simulink model "a2e1"  (R2020a)
settings: Solver=VariableStepAuto  StartTime=0.0  StopTime=400000  RelTol=1e-3
settings Model: EnablePacing=on  PacingRate=6  Creator=mumun  LastModifiedBy=mumun

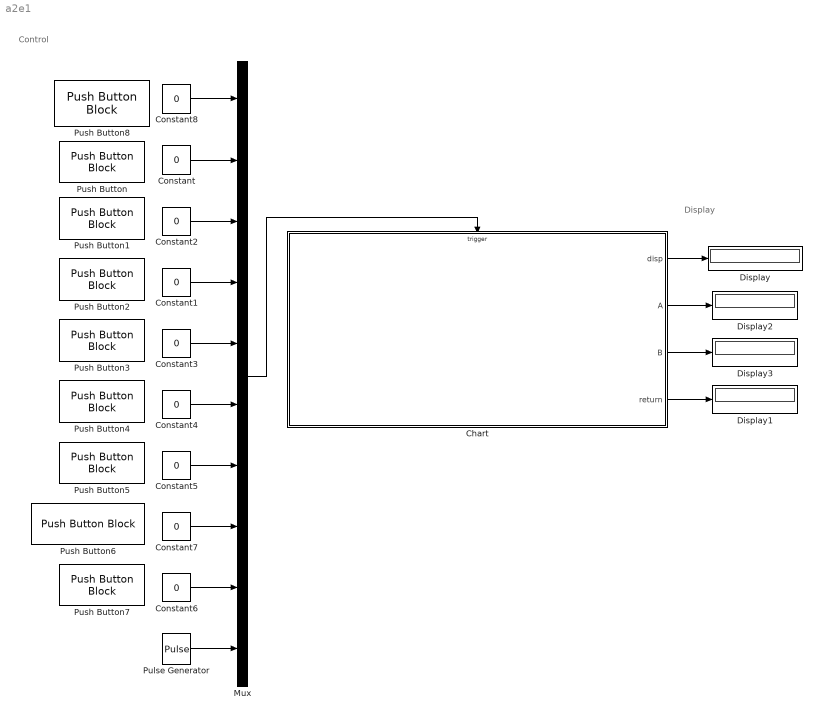
== system a2e1 ==
  note: Display
  note: Control
  Chart : Stateflow chart  TreatAsAtomicUnit=on
  Constant{,1..8} (9 alike) : Constant  Value=0
  Display{,1..3} (4 alike) : Display
  Mux : Mux  Inputs=10
  Pulse Generator : DiscretePulseGenerator  PulseType=Time based  Period=1  PulseWidth=5
  Push Button : PushButtonBlock  ButtonText=1kr
  Push Button1 : PushButtonBlock  ButtonText=5kr
  Push Button2 : PushButtonBlock  ButtonText=10kr
  Push Button3 : PushButtonBlock  ButtonText=order
  Push Button4 : PushButtonBlock  ButtonText=option_A
  Push Button5 : PushButtonBlock  ButtonText=option_B
  Push Button6 : PushButtonBlock  ButtonText=insert_more_money
  Push Button7 : PushButtonBlock  ButtonText=finish
  Push Button8 : PushButtonBlock  ButtonText=Start_Button
  wires:
  Mux/1 -> Chart/Trigger
  Chart/1(disp) -> Display/1
  Constant8/1 -> Mux/1
  Constant/1 -> Mux/2
  Constant2/1 -> Mux/3
  Constant1/1 -> Mux/4
  Constant3/1 -> Mux/5
  Constant4/1 -> Mux/6
  Constant5/1 -> Mux/7
  Constant7/1 -> Mux/8
  Constant6/1 -> Mux/9
  Chart/3(B) -> Display3/1
  Pulse Generator/1 -> Mux/10
  Chart/4(return) -> Display1/1
  Chart/2(A) -> Display2/1

== stateflow chart a2e1/Chart ==
  settings: executeAtInitialization=1  initializeOutput=1
  state coininsert
    du: disp= 'Insert coin';
    on one_kr: coin_count=coin_count+1;
    on five_kr: coin_count=coin_count+5;
    on ten_kr: coin_count=coin_count+10;
  state Idle
    en, du: disp= 'Welcome'; coin_count=0;
    en: A=0; B=0;
  state order
    du: disp= 'Choose option';
  state deliverA
    en: coin_count = coin_count-8;
    du:return=coin_count;
    du: disp= 'Product A delivered';
    du: A=A+1;
  state optionA
    du: disp= 'Option A selected';
  state optionB
    du: disp= 'Option B selected';
  state deliverB
    en: coin_count = coin_count-6;
    du: return=coin_count;
    du: disp= 'Product B delivered ';
    du: B=B+1;
  (default) -> Idle
  coininsert -> order [order 1] : order
  Idle -> coininsert : Start_signal
  deliverB -> order [order 3] : order
  deliverA -> order [order 3] : order
  order -> optionA [order 2] : option_A
  order -> optionB [order 1] : option_B
  deliverB -> Idle [order 2] : Finish
  deliverA -> Idle [order 1] : Finish
  coininsert -> Idle [order 2] : Finish{return=coin_count}
  deliverB -> coininsert [order 1] : insert_more_money
  deliverA -> coininsert [order 2] : insert_more_money
  optionA -> coininsert [order 1] : [coin_count<8]{disp='Sorry'}
  optionB -> coininsert [order 1] : [coin_count<6]{disp='Sorry'}
  optionB -> deliverB [order 2] : [coin_count>=6]
  optionA -> deliverA [order 2] : [coin_count>=8]
  data: disp output string; A output; B output; return output; coin_count local int8
  events: Start_signal input RISING_EDGE_EVENT; one_kr input RISING_EDGE_EVENT; five_kr input RISING_EDGE_EVENT; ten_kr input RISING_EDGE_EVENT; order input RISING_EDGE_EVENT; option_A input RISING_EDGE_EVENT; option_B input RISING_EDGE_EVENT; insert_more_money input RISING_EDGE_EVENT; Finish input RISING_EDGE_EVENT; pulse input RISING_EDGE_EVENT
